simulink model "KalmanTeste1"  (R2021a)
settings: Solver=VariableStepAuto  StartTime=0.0  StopTime=24  RelTol=1e-3
values from neighbouring files (symbols this model uses):
  N = 0    [parse31.m]    (also in parse3e4_kalmanSemBias.m)
  Rpitch = 0.5*Qpitch    (= 0.0071)    [parse31.m]    (also in parse3e4_kalmanComBias.m = 0.011; parse3e4_kalmanSemBias.m = 0.0146)
  Rroll = 2*Qroll    (= 0.15)    [parse31.m]    (also in parse3e4_kalmanComBias.m = 1.575; parse3e4_kalmanSemBias.m = 0.0465)
undefined symbols (not defined in the file or in its folder): Continuous, Time
libraries: ctrlSharedLib x2, simulink_extras x2
settings Model: Creator=Pedrus  LastModifiedBy=Pedrus

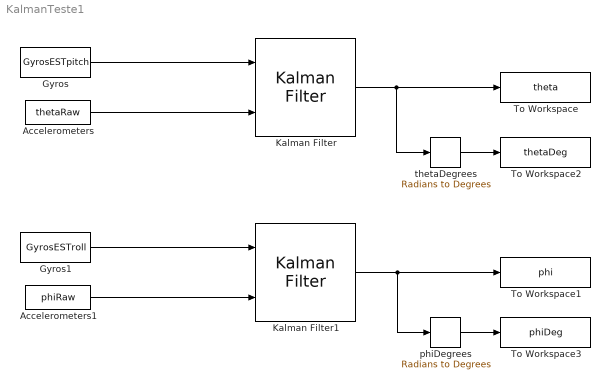
== system KalmanTeste1 ==
  Accelerometers : FromWorkspace  VariableName=thetaRaw
  Accelerometers1 : FromWorkspace  VariableName=phiRaw
  Gyros : FromWorkspace  VariableName=GyrosESTpitch
  Gyros1 : FromWorkspace  VariableName=GyrosESTroll
  Kalman Filter : ctrlSharedLib/Kalman Filter  TimeDomain=Continuous-Time  UseCurrentEstimator=on  ModelSource=LTI State-Space Variable  ModelSourceVariable=kalmfpitch  A=0.95  B=1  C=1  D=0  NumberOfStates=1  NumberOfInputs=1  NumberOfOutputs=1  InitialEstimateSource=Dialog  X0=0  P0=10  UseK=off  UseGH=off  NumberOfProcessNoiseInputs=1  G=1  TimeInvariantG=on  H=0  TimeInvariantH=on  Q=Qpitch  TimeInvariantQ=on  R=Rpitch  TimeInvariantR=on  N=N  TimeInvariantN=on  AddInputPort=on  AddEnablePort=off  OutputEstimatedY=off  OutputP=off  Ts=-1
  Kalman Filter1 : ctrlSharedLib/Kalman Filter  TimeDomain=Continuous-Time  UseCurrentEstimator=on  ModelSource=LTI State-Space Variable  ModelSourceVariable=kalmfroll  A=0.95  B=1  C=1  D=0  NumberOfStates=1  NumberOfInputs=1  NumberOfOutputs=1  InitialEstimateSource=Dialog  X0=0  P0=10  UseK=off  UseGH=off  NumberOfProcessNoiseInputs=1  G=1  TimeInvariantG=on  H=0  TimeInvariantH=on  Q=Qroll  TimeInvariantQ=on  R=Rroll  TimeInvariantR=on  N=N  TimeInvariantN=on  AddInputPort=on  AddEnablePort=off  OutputEstimatedY=off  OutputP=off  Ts=-1
  To Workspace : ToWorkspace  VariableName=theta  SaveFormat=Timeseries  SampleTime=-1
  To Workspace1 : ToWorkspace  VariableName=phi  SaveFormat=Timeseries  SampleTime=-1
  To Workspace2 : ToWorkspace  VariableName=thetaDeg  SaveFormat=Timeseries  SampleTime=-1
  To Workspace3 : ToWorkspace  VariableName=phiDeg  SaveFormat=Timeseries  SampleTime=-1
  phiDegrees : simulink_extras/Transformations/Radians to Degrees
  thetaDegrees : simulink_extras/Transformations/Radians to Degrees
  wires:
  Gyros/1 -> Kalman Filter/1
  Kalman Filter/1 -> thetaDegrees/1, To Workspace/1
  Accelerometers/1 -> Kalman Filter/2
  Accelerometers1/1 -> Kalman Filter1/2
  Kalman Filter1/1 -> phiDegrees/1, To Workspace1/1
  Gyros1/1 -> Kalman Filter1/1
  thetaDegrees/1 -> To Workspace2/1
  phiDegrees/1 -> To Workspace3/1
